simulink model "DC_Motor_control_speed_Direction_Push_Button"  (R2024a)
settings: Solver=FixedStepDiscrete  StartTime=0.0  StopTime=inf  FixedStep=1e-3  RelTol=1e-3  EnableMultiTasking=on
libraries: arduinolib x6
settings Model: ExtModeTrigDuration=2  Creator=DELL  LastModifiedBy=DELL
settings SolverCC: AutoInsertRateTranBlk=on
settings OptimizationCC: EnhancedBackFolding=on  PassReuseOutputArgsAs=Individual arguments  ZeroExternalMemoryAtStartup=off  ZeroInternalMemoryAtStartup=off  MaxStackSize=64  OptimizeBlockOrder=speed  DifferentSizesBufferReuse=on  OptimizationCustomize=off  EfficientTunableParamExpr=on
settings DebuggingCC: ParameterTunabilityLossMsg=error
settings HardwareCC: ProdBitPerInt=16  ProdBitPerPointer=16  ProdBitPerSizeT=16  ProdBitPerPtrDiffT=16  ProdLargestAtomicFloat=None  ProdWordSize=8  ProdHWDeviceType=Atmel->AVR
settings SFSimCC: MATLABDynamicMemAlloc=off
settings RTWCC: Description=Embedded Coder  SystemTargetFile=ert.tlc  HardwareBoard=Arduino Uno  TemplateMakefile=ert_default_tmf  Toolchain=Arduino AVR  BuildConfiguration=Faster Runs
settings CodeAppCC: ForceParamTrailComments=on  IgnoreCustomStorageClasses=off  OperatorAnnotations=on  SimulinkDataObjDesc=on  SFDataObjDesc=on  InsertBlockDesc=on
settings ERTTargetCC: SupportContinuousTime=on  SupportVariableSizeSignals=on  ExtModeTransport=3  ExtModeStaticAlloc=on  ExtModeAutomaticAllocSize=off  ExtModeStaticAllocSize=250  ExtModeMexFile=ext_xcp  ExtModeIntrfLevel=Level2 - Open

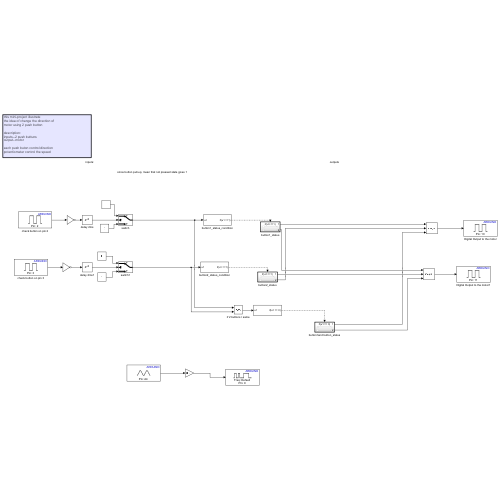
[thumbnail: Simulink's stored preview of the top-level diagram]
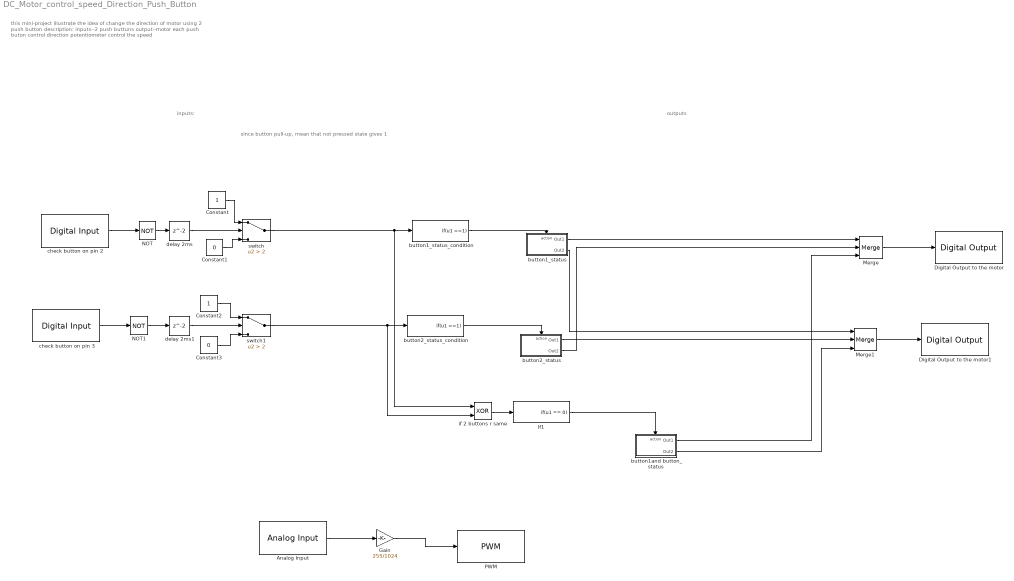
== system DC_Motor_control_speed_Direction_Push_Button ==
  note: outputs
  note: inputs:
  note: this mini-project illustrate
      | the idea of change the direction of
      | motor using 2 push button
      |
      | description:
      | inputs--2 push buttuns
      | output--motor
      |
      | each push buton control direction
      | potentiometer control the speed
  note: since button pull-up, mean that not pressed state gives 1
  Analog Input : arduinolib/Analog Input  pinNumber=4  ReadResultsOnly=off  ConversionTriggerSource=Software  ExternalTriggerType=uint32( 0 )  OutputDataType=uint16  EnableConversionCompleteNotify=off  EnableOuputStatus=off  SampleTime=-1  blockPlatform=arduino
  Constant : Constant
  Constant1 : Constant  Value=0
  Constant2 : Constant
  Constant3 : Constant  Value=0
  Digital Output to the motor : arduinolib/Digital Output  pinNumber=10  Direction=output  blockPlatform=arduino
  Digital Output to the motor1 : arduinolib/Digital Output  pinNumber=11  Direction=output  blockPlatform=arduino
  Gain : Gain  Gain=255/1024
  If1 : If  IfExpression=u1 == 0  ShowElse=off
  Merge : Merge  Inputs=3
  Merge1 : Merge  Inputs=3
  NOT : Logic  Operator=NOT  IconShape=distinctive  AllPortsSameDT=off  OutDataTypeStr=boolean
  NOT1 : Logic  Operator=NOT  IconShape=distinctive  AllPortsSameDT=off  OutDataTypeStr=boolean
  PWM : arduinolib/PWM  pinNumber=9  frequencyType=Default  desiredFrequency=490.2  achievableFrequency=490.2
  button1_status : Subsystem  TreatAsAtomicUnit=on
  button1_status_condition : If  IfExpression=u1 ==1  ShowElse=off
  button1and button_status : Subsystem  TreatAsAtomicUnit=on
  button2_status : Subsystem  TreatAsAtomicUnit=on
  button2_status_condition : If  IfExpression=u1 ==1  ShowElse=off
  check button on pin 2 : arduinolib/Digital Input  pinNumber=2  mode=Input Pullup  Direction=input  SampleTime=0.1  blockPlatform=arduino
  check button on pin 3 : arduinolib/Digital Input  pinNumber=3  mode=Input Pullup  Direction=input  SampleTime=0.1  blockPlatform=arduino
  delay 2ms : Delay
  delay 2ms1 : Delay
  if 2 buttons r same : Logic  Operator=XOR  AllPortsSameDT=off  OutDataTypeStr=boolean
  switch : Switch  Criteria=u2 > Threshold  Threshold=2  SaturateOnIntegerOverflow=off  InputSameDT=off
  switch1 : Switch  Criteria=u2 > Threshold  Threshold=2  SaturateOnIntegerOverflow=off  InputSameDT=off
  wires:
  check button on pin 2/1 -> NOT/1
  check button on pin 3/1 -> NOT1/1
  Analog Input/1 -> Gain/1
  Gain/1 -> PWM/1
  NOT/1 -> delay 2ms/1
  delay 2ms1/1 -> switch1/2
  delay 2ms/1 -> switch/2
  Merge/1 -> Digital Output to the motor/1
  Constant/1 -> switch/1
  Constant1/1 -> switch/3
  Constant2/1 -> switch1/1
  Constant3/1 -> switch1/3
  button1_status_condition/1 -> button1_status/Action
  Merge1/1 -> Digital Output to the motor1/1
  switch/1 -> if 2 buttons r same/1, button1_status_condition/1
  button2_status_condition/1 -> button2_status/Action
  switch1/1 -> if 2 buttons r same/2, button2_status_condition/1
  button1_status/1(Out1) -> Merge/1
  button1_status/2(Out2) -> Merge1/1
  button2_status/1(Out1) -> Merge1/2
  button2_status/2(Out2) -> Merge/2
  if 2 buttons r same/1 -> If1/1
  If1/1 -> button1and button_status/Action
  button1and button_status/1(Out1) -> Merge/3
  button1and button_status/2(Out2) -> Merge1/3
  NOT1/1 -> delay 2ms1/1

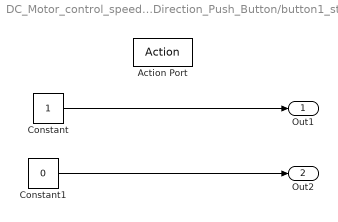
== system DC_Motor_control_speed_Direction_Push_Button/button1_status ==
  Action Port : ActionPort  ActionPortLabel=if(u1 ==1)
  Constant : Constant  OutDataTypeStr=boolean
  Constant1 : Constant  Value=0  OutDataTypeStr=boolean
  Out1 : Outport
  Out2 : Outport  Port=2
  wires:
  Constant/1 -> Out1/1
  Constant1/1 -> Out2/1

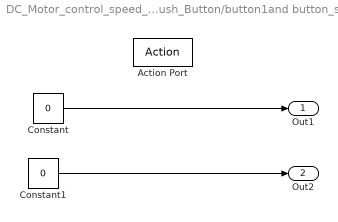
== system DC_Motor_control_speed_Direction_Push_Button/button1and button_status ==
  Action Port : ActionPort  ActionPortLabel=if(u1 == 0)
  Constant : Constant  Value=0  OutDataTypeStr=boolean
  Constant1 : Constant  Value=0  OutDataTypeStr=boolean
  Out1 : Outport
  Out2 : Outport  Port=2
  wires:
  Constant/1 -> Out1/1
  Constant1/1 -> Out2/1

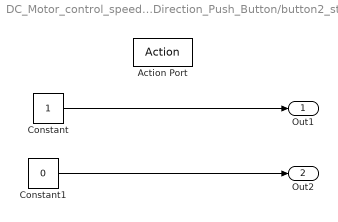
== system DC_Motor_control_speed_Direction_Push_Button/button2_status ==
  Action Port : ActionPort  ActionPortLabel=if(u1 ==1)
  Constant : Constant  OutDataTypeStr=boolean
  Constant1 : Constant  Value=0  OutDataTypeStr=boolean
  Out1 : Outport
  Out2 : Outport  Port=2
  wires:
  Constant1/1 -> Out2/1
  Constant/1 -> Out1/1
